simulink subsystem "Estimator"  (R2025a)
settings: Solver=VariableStepAuto  StartTime=0.0  StopTime=10.0  RelTol=1e-3
undefined symbols (not defined in the file): gyro_bias_rw, gyro_sigma, star_sigma, Ts_base
settings Model: Creator=Jackt  LastModifiedBy=Jackt

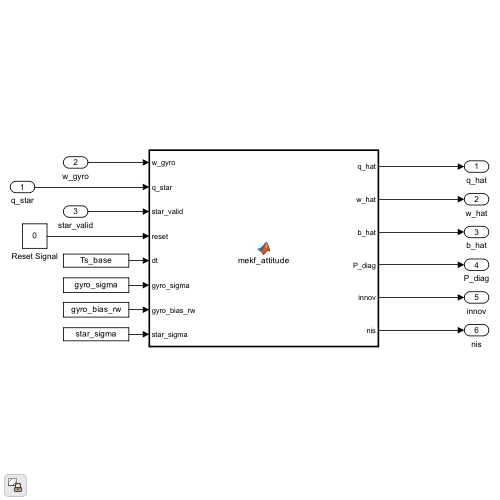
[thumbnail: Simulink's stored preview of the top-level diagram]
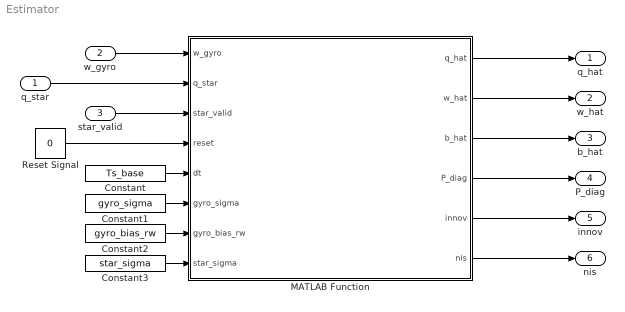
== system Estimator ==
  q_star : Inport
  w_gyro : Inport  Port=2
  star_valid : Inport  Port=3
  Constant : Constant  Value=Ts_base  VectorParams1D=off
  Constant1 : Constant  Value=gyro_sigma  VectorParams1D=off
  Constant2 : Constant  Value=gyro_bias_rw  VectorParams1D=off
  Constant3 : Constant  Value=star_sigma  VectorParams1D=off
  MATLAB Function : MATLAB Function  TreatAsAtomicUnit=on
  Reset Signal : Constant  Value=0
  q_hat : Outport
  w_hat : Outport  Port=2
  b_hat : Outport  Port=3
  P_diag : Outport  Port=4
  innov : Outport  Port=5
  nis : Outport  Port=6
  wires:
  MATLAB Function/1(q_hat) -> q_hat/1
  MATLAB Function/2(w_hat) -> w_hat/1
  MATLAB Function/3(b_hat) -> b_hat/1
  MATLAB Function/4(P_diag) -> P_diag/1
  MATLAB Function/5(innov) -> innov/1
  MATLAB Function/6(nis) -> nis/1
  w_gyro/1 -> MATLAB Function/1(w_gyro)
  q_star/1 -> MATLAB Function/2(q_star)
  star_valid/1 -> MATLAB Function/3(star_valid)
  Reset Signal/1 -> MATLAB Function/4(reset)
  Constant/1 -> MATLAB Function/5(dt)
  Constant1/1 -> MATLAB Function/6(gyro_sigma)
  Constant2/1 -> MATLAB Function/7(gyro_bias_rw)
  Constant3/1 -> MATLAB Function/8(star_sigma)

== matlab function Estimator/MATLAB Function ==
  data: q_hat output; w_hat output; b_hat output; P_diag output; innov output; nis output; w_gyro input; q_star input; star_valid input; reset input; dt input; gyro_sigma input; gyro_bias_rw input; star_sigma input
function [q_hat, w_hat, b_hat, P_diag, innov, nis] = mekf_attitude(w_gyro, q_star, star_valid, reset, dt, gyro_sigma, gyro_bias_rw, star_sigma)
%MEKF_ATTITUDE Error state MEKF for attitude and gyro bias.

%Force input shapes
w_gyro = reshape(w_gyro, [3 1]);
q_star = reshape(q_star, [4 1]);

%Initialize persistent filter states
persistent q b P is_init q_prev star_valid_prev
if isempty(is_init) || reset
    q = [1; 0; 0; 0];
    b = zeros(3,1);
    P = diag([ (deg2rad(5))^2*ones(1,3), (deg2rad(0.5))^2*ones(1,3) ]);
    q_prev = q;
    star_valid_prev = 0;   % <-- DOUBLE (0/1), codegen-safe
    is_init = true;
end

%Normalize q_star
q_star = q_star / max(norm(q_star), 1e-12);

%Build covariance matrices
R = (star_sigma^2) * eye(3);
Qd = diag([ (gyro_sigma^2)*dt * ones(1,3), ...
            (gyro_bias_rw^2)*dt * ones(1,3) ]);

%Compute bias corrected body rate
w = w_gyro - b;

%Propagate nominal quaternion state
dq = rotvec_to_quat(0.5*w*dt);
q = quatmultiply_sf(q, dq);
q = q / max(norm(q), 1e-12);

%Enforce quaternion sign continuity
if dot(q, q_prev) < 0
    q = -q;
end
q_prev = q;

%Propagate error state covariance
Wx = skew(w);
F = [ eye(3) - Wx*dt,   -eye(3)*dt;
      zeros(3),         eye(3) ];
P = F*P*F.' + Qd;
P = 0.5*(P + P.');

%Initialize measurement outputs
innov = zeros(3,1);
nis = 0;

%Rising-edge detect star_valid
sv = 0;
if star_valid ~= 0
    sv = 1;
end
do_update = (sv == 1) && (star_valid_prev == 0);
star_valid_prev = sv;

%Apply star tracker measurement update
if do_update
    %Align measurement sign with estimate
    if dot(q_star, q) < 0
        q_star = -q_star;
    end

    %Right-invariant innovation quaternion
    % q_e = inv(q_hat) ⊗ q_star
    q_inv = [q(1); -q(2:4)];
    q_e = quatmultiply_sf(q_inv, q_star);
    q_e = q_e / max(norm(q_e), 1e-12);

    %Use shortest rotation for innovation
    if q_e(1) < 0
        q_e = -q_e;
    end

    %Log-map innovation
    y = quat_log_sf(q_e);
    innov = y;

    %Build measurement Jacobian
    H = [eye(3), zeros(3)];

    %Compute Kalman gain
    S = H*P*H.' + R;
    K = (P*H.') / S;

    %Compute correction for attitude error and bias
    dx = K*y;
    dtheta = dx(1:3);
    db = dx(4:6);

    %Update covariance with Joseph form
    I6 = eye(6);
    P = (I6 - K*H)*P*(I6 - K*H).' + K*R*K.';
    P = 0.5*(P + P.');

    %Inject bias correction
    b = b + db;

    %Inject attitude correction into quaternion
    dq_inj = rotvec_to_quat(0.5*dtheta);
    q = quatmultiply_sf(q, dq_inj);
    q = q / max(norm(q), 1e-12);

    %Enforce quaternion sign continuity after update
    if dot(q, q_prev) < 0
        q = -q;
    end
    q_prev = q;

    %Compute normalized innovation squared
    nis = y.'*(S\y);
end

%Package estimator outputs
q_hat = q;
b_hat = b;
w_hat = w_gyro - b;
P_diag = diag(P);

end

function S = skew(w)
%SKEW Returns the skew symmetric matrix for cross products.
S = [   0   -w(3)  w(2);
      w(3)    0   -w(1);
     -w(2)  w(1)    0  ];
end

function q = rotvec_to_quat(v)
%ROTVEC_TO_QUAT Converts a rotation vector to a quaternion scalar first.
theta = norm(v);
if theta < 1e-12
    q = [1; 0; 0; 0];
else
    u = v/theta;
    q = [cos(theta); u*sin(theta)];
end
end

function r = quat_log_sf(q)
%QUAT_LOG_SF Robust log-map from unit quaternion (scalar-first) to rotvec.
q = q / max(norm(q), 1e-12);
if q(1) < 0
    q = -q; %shortest rotation
end
w = max(-1, min(1, q(1)));
v = q(2:4);
nv = norm(v);
if nv < 1e-8
    r = 2*v; %small-angle limit
else
    ang = 2*atan2(nv, w);
    r = (ang/nv) * v;
end
end

function q = quatmultiply_sf(a, b)
%QUATMULTIPLY_SF Quaternion multiply scalar first.
w1 = a(1); x1 = a(2); y1 = a(3); z1 = a(4);
w2 = b(1); x2 = b(2); y2 = b(3); z2 = b(4);
q = [ w1*w2 - x1*x2 - y1*y2 - z1*z2;
      w1*x2 + x1*w2 + y1*z2 - z1*y2;
      w1*y2 - x1*z2 + y1*w2 + z1*x2;
      w1*z2 + x1*y2 - y1*x2 + z1*w2 ];
end
